simulink model "inductive_sensor"  (R2021a)
settings: Solver=VariableStepAuto  StartTime=0.0  StopTime=0.1  RelTol=1e-3
libraries: simulink x2, simulink_extras x1
settings Model: Creator=kjartan  LastModifiedBy=kjartan

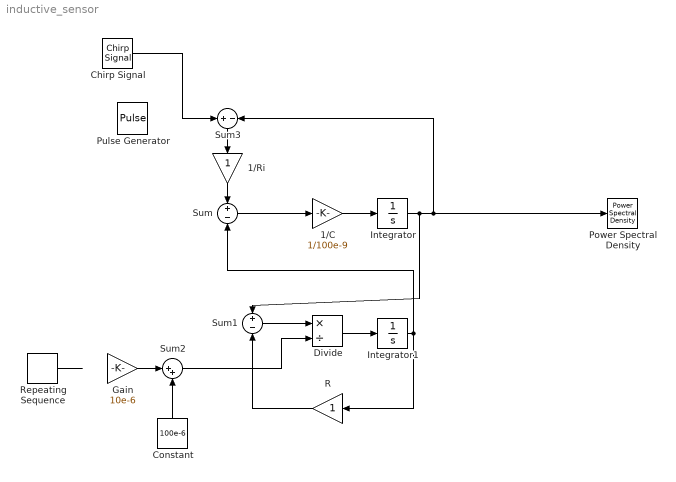
== system inductive_sensor ==
  1/C : Gain  Gain=1/100e-9
  1/Ri : Gain
  Chirp Signal : simulink/Sources/Chirp Signal  f1=0.1  T=1  f2=50e3
  Constant : Constant  Value=100e-6
  Divide : Product  Inputs=*/
  Gain : Gain  Gain=10e-6
  Integrator : Integrator
  Integrator1 : Integrator
  Power Spectral Density : simulink_extras/Additional Sinks/Power Spectral Density  npts=128  fftpts=512  HowOften=64  sampleT=1/200e3
      settings: SourceProductBaseCode=SL
  Pulse Generator : DiscretePulseGenerator  PulseType=Time based  Period=1/50e3  PulseWidth=50
  R : Gain
  Repeating Sequence : simulink/Sources/Repeating Sequence  rep_seq_t=[0 2]  rep_seq_y=[0 5]
  Sum : Sum  Inputs=+|-
  Sum1 : Sum  Inputs=+|-
  Sum2 : Sum  Inputs=|++
  Sum3 : Sum  Inputs=+|-
  wires:
  1/C/1 -> Integrator/1
  Sum/1 -> 1/C/1
  Integrator/1 -> Sum3/2, Power Spectral Density/1, Sum1/1
  Divide/1 -> Integrator1/1
  Sum1/1 -> Divide/1
  Chirp Signal/1 -> Sum3/1
  Repeating Sequence/1 -> ?
  Constant/1 -> Sum2/2
  Sum2/1 -> Divide/2
  Sum3/1 -> 1/Ri/1
  1/Ri/1 -> Sum/1
  Integrator1/1 -> Sum/2, R/1
  R/1 -> Sum1/2
  Gain/1 -> Sum2/1
